simulink model "PMSM_FOC_Average_Inveter"  (R2020b)
settings: Solver=FixedStepAuto  StartTime=0.0  StopTime=10  FixedStep=Fixed_Step_Size  RelTol=1e-3
model workspace (MAT data in the model file):
  wc : Simulink.Parameter (value not decoded)
values from neighbouring files (symbols this model uses):
  Angle = 1.0    [Hall_HSMO_FOC_Data.sldd]    (also in Hall_SMO_FOC_Data.sldd)
  Angle_offset = 0.1985    [Hall_HSMO_FOC_Data.sldd]    (also in Hall_SMO_FOC_Data.sldd)
  Cosine_table = 1.0 0.99999529 0.99999058 0.99998587 0.99998116 0.99996704 0.99995291 0.99993885 0.99992472 0.99990118 0.99987763 0.99985409 0.9998306 0.99979764 0.99976468 0.99973178 0.99969882 0.99965644 0.99961412 0.99957174 0.99952942 0.99947762 0.99942589 0.99937415 0.99932235 0.9992612 0.99920005 0.99913889 0.99907768 0.99900717 0.99893659 0.99886602 0.99879545 0.99871546 0.99863547 0.99855554 0.99847555 0.    [Hall_HSMO_FOC_Data.sldd]    (also in Hall_SMO_FOC_Data.sldd)
  Fixed_Step_Size = 2.5E-5    [Hall_HSMO_FOC_Data.sldd]    (also in Hall_SMO_FOC_Data.sldd = 1.0E-5
  Flux = 0.0109    [G474_FOC_HSMO.sldd]    (also in Hall_HSMO_FOC_Data.sldd = 0.00529276
  FluxWeak_Enable = 0.0    [Hall_HSMO_FOC_Data.sldd]    (also in Hall_SMO_FOC_Data.sldd)
  FluxWeak_Idref_max = 0.0    [Hall_HSMO_FOC_Data.sldd]    (also in Hall_SMO_FOC_Data.sldd)
  FluxWeak_Idref_min = -200.0    [Hall_HSMO_FOC_Data.sldd]    (also in Hall_SMO_FOC_Data.sldd)
  FluxWeak_Ki = 50.0    [Hall_HSMO_FOC_Data.sldd]    (also in Hall_SMO_FOC_Data.sldd)
  FluxWeak_Kp = 1.2    [Hall_HSMO_FOC_Data.sldd]    (also in Hall_SMO_FOC_Data.sldd)
  ID_Ki = 450.0    [Hall_HSMO_FOC_Data.sldd]    (also in Hall_SMO_FOC_Data.sldd = 0.8
  ID_Kp = 0.4    [Hall_HSMO_FOC_Data.sldd]    (also in Hall_SMO_FOC_Data.sldd = 3.2
  IQ_Ki = 450.0    [Hall_HSMO_FOC_Data.sldd]    (also in Hall_SMO_FOC_Data.sldd = 0.32
  IQ_Kp = 0.45    [Hall_HSMO_FOC_Data.sldd]    (also in Hall_SMO_FOC_Data.sldd = 3.3
  Ld = 0.000195185    [G474_FOC_HSMO.sldd]    (also in Hall_HSMO_FOC_Data.sldd = 0.0004
  Lq = 0.000195185    [G474_FOC_HSMO.sldd]    (also in Hall_HSMO_FOC_Data.sldd = 0.00045
  MTPA_id_table = 0.22889 0.23462678 0.23770036 0.2381243 0.23591207 0.23107713 0.2236329 0.21359272 0.20096992 0.18577772 0.16802935 0.14773798 0.12491672 0.099578641 0.071736768 0.041404068 0.0085934745 -0.026682133 -0.064409919 -0.10457709 -0.14717092 -0.1921787 -0.2395878 -0.28938559 -0.34155953 -0.39609709 -0.45298585 -0.51221335 -0.57376724 -0.63763517 -0.70380485 -0.77226412 -0.84300071 -0.91600245 -0.991257    [Hall_HSMO_FOC_Data.sldd]    (also in Hall_SMO_FOC_Data.sldd)
  MTPA_iq_table = -1.0417 -0.16083497 0.71926296 1.5985928 2.4771533 3.3549435 4.2319627 5.1082091 5.9836826 6.8583813 7.732305 8.6054525 9.4778223 10.349415 11.220228 12.090261 12.959513 13.827983 14.69567 15.562573 16.428694 17.294027 18.158575 19.022335 19.885307 20.747492 21.608887 22.469492 23.329306 24.188328 25.046556 25.903992 26.760633 27.616482 28.471533 29.325788 30.179247 31.031908 31.883772 32.734837 3    [Hall_HSMO_FOC_Data.sldd]    (also in Hall_SMO_FOC_Data.sldd)
  MTPA_Te_Max = 800.0    [Hall_HSMO_FOC_Data.sldd]    (also in Hall_SMO_FOC_Data.sldd)
  MTPA_Te_Min = 0.0    [Hall_HSMO_FOC_Data.sldd]    (also in Hall_SMO_FOC_Data.sldd)
  Over_modulation = 0.0    [Hall_HSMO_FOC_Data.sldd]    (also in Hall_SMO_FOC_Data.sldd)
  Pole_Pairs = 2.0    [Hall_HSMO_FOC_Data.sldd]    (also in Hall_SMO_FOC_Data.sldd)
  PWM_Frequency = 10000.0    [Hall_HSMO_FOC_Data.sldd]    (also in Hall_SMO_FOC_Data.sldd)
  Sine_table = 0.0 0.0015339879 0.0030679768 0.0046019657 0.0061359555 0.0076698866 0.0092038177 0.010737749 0.012271681 0.013805497 0.015339312 0.016873131 0.018406944 0.019940587 0.021474229 0.023007872 0.024541514 0.026074925 0.027608337 0.029141748 0.03067516 0.032208283 0.033741407 0.035274528 0.036807653 0.038340431 0.039873205 0.04140598 0.042938754 0.04447113 0.046003502 0.047535874 0.049068246 0.0506001    [Hall_HSMO_FOC_Data.sldd]    (also in Hall_SMO_FOC_Data.sldd)
  Speed_Ki = 0.633    [Hall_HSMO_FOC_Data.sldd]    (also in Hall_SMO_FOC_Data.sldd)
  Speed_Kp = 0.0867    [Hall_HSMO_FOC_Data.sldd]    (also in Hall_SMO_FOC_Data.sldd = 0.0267
  Speed_PI_OutputMax = 6.0    [Hall_HSMO_FOC_Data.sldd]    (also in Hall_SMO_FOC_Data.sldd = 5.0
  Speed_PI_OutputMin = -6.0    [Hall_HSMO_FOC_Data.sldd]    (also in Hall_SMO_FOC_Data.sldd = -5.0
  TorqueMode = 0.0    [Hall_HSMO_FOC_Data.sldd]    (also in Hall_SMO_FOC_Data.sldd)
undefined symbols (not defined in the file or in its folder): DiscIntNeverNeededParam, inverter, sigbuilder_block, SVPWM
libraries: simulink x7, pid_lib x1, mcbplantlib x1, autolibpmsminterior x1
(part 3 of 3)

== stateflow chart PMSM_FOC_Average_Inveter/Motor_Control/Motor_Control_Function/SYM_State_10ms/Traction_SYM ==
  state Drive
    en:
    stSysCtlDes = Drive;
    SYM_Current_State=0;
    state SYM_InvrStM
      en,du:
      state Second_State
        state Init
          en,du:
          flgTranDrvInit=1;
        state DrvInit
          en,du:
          flgTranDrvInitToCal=1;
        state Calibration
          state MoCSop
            en,du:
            stSysCtlDes=MoCSop;
          state SensCalFW
            en,du:
            stSysCtlDes=SensCalFW
          state TestPulse
            en,du:
            stSysCtlDes=TestPulse
          (default) -> MoCSop
          SensCalFW -> TestPulse : [flgTranSnsrCalToTestPls]
          MoCSop -> SensCalFW : [flgTranMoCSOPToSnsrCal]
        state FreeWheel
          en,du:
          stSysCtlDes=FreeWheel;
        state alOffsetCalFW
          en,du:
          stSysCtlDes=alOffsetCalFW;
        state Standby
          en,du:
          stSysCtlDes=Standby;
          SYM_flgRunRea=1;
          Standby -> (junction 246) [order 1]
          (junction 246) -> Standby : [stDrvCtlDes==Run]{flgTranStbToCtrl=1}
        state alOffsetCalAcc
          en,du:
          stSysCtlDes=alOffsetCalAcc;
        state Run
          en,du:
          stSysCtlDes=Run;
          flgTranStbToCtrl=1;
          SYM_flgRunRea=0;
          exit:
          SYM_flgRunRea=1;
          Run -> (junction 243) [order 1]
          (junction 243) -> Run : [stDrvCtlDes==Standby]{flgTranStbToCtrl=0}
        (default) -> Init
        (junction 145) -> Init [order 1] : [~flgStbRea]
        Init -> DrvInit : [flgTranDrvInit]
        FreeWheel -> (junction 145) : [~flgTranToFW]
        (junction 145) -> Standby [order 2] : [flgStbRea]
        DrvInit -> Run [order 3] : [flgTranDrvInitToCal ...
            | &&stDrvCtlDes== Run]
        DrvInit -> Standby [order 2] : [flgTranDrvInitToCal ...
            | &&stDrvCtlDes== Standby]
        DrvInit -> Calibration [order 1] : [flgTranDrvInitToCal ...
            | &&stDrvCtlDes== Calibration]
        Second_State -> FreeWheel [order 1] : [flgTranToFW]
        Calibration -> Run [order 1] : [flgTranMoCSOPToRun ...
            | && stDrvCtlDes== Run ]
        Calibration -> Standby [order 2] : [flgTranCalToStb]
        alOffsetCalFW -> Standby [order 1] : [stDrvCtlDes~=alOffsetCalFW]
        Standby -> alOffsetCalFW [order 2] : [stDrvCtlDes==alOffsetCalFW]
        alOffsetCalFW -> alOffsetCalAcc [order 2] : [stDrvCtlDes==alOffsetCalAcc]
        alOffsetCalAcc -> alOffsetCalFW [order 1] : [stDrvCtlDes==alOffsetCalFW]
        Run -> Standby [order 1] : [~flgTranStbToCtrl]
        Standby -> Run [order 1] : [flgTranStbToCtrl]
        Standby -> alOffsetCalAcc [order 3] : [stDrvCtlDes==alOffsetCalAcc]
        alOffsetCalAcc -> Standby [order 2] : [stDrvCtlDes~=alOffsetCalAcc]
      state Failure
        en,du:
        stSysCtlDes=FreeWheel;
      state Discharge
        en,du:
        stSysCtlDes=Discharge;
      (default) -> Second_State
      Failure -> (junction 145) : [flgTranErrToStb]
      Discharge -> (junction 145) : [~flgTranDcha]
      Second_State -> Failure [order 1] : [flgTranToErr]
      SYM_InvrStM -> Discharge [order 1] : [flgTranDcha]
    state SYM_Invrlnp
      en:SYM_Current_State=10;
      state SYM_Invrlnp_Check
        en:SYM_Current_State=11;
      (default) -> SYM_Invrlnp_Check
    (junction 258) -> Drive
    SYM_Invrlnp -> (junction 258) : [ISC_bT15==0]{flgAllwDrv=0}
    SYM_InvrStM -> (junction 258) [order 1] : [ISC_bT15==0]{flgAllwDrv=0}
    (default) -> SYM_Invrlnp
    SYM_Invrlnp_Check -> SYM_InvrStM : [flgCmpIMsg ...
        | && ISC_UdcLnkFlt>10 ...
        | && ISC_UdcLnkFlt<450 ...
        | && ISC_bT15 ...
        | && stSysCtlDes==Drive]
  state SYM_OperInp
    en,du:
    flgAllwDrv=0;
    SYM_Current_State=SYM_OperInp;
  state PreDrive
    en:
    stSysCtlDes = PreDrive;
    flgAllwDrv=1;
    %tiPreActvTi++;
    SYM_Current_State=PreDrive;
  state PostDrive
    en:
    stSysCtlDes=PostDrive;
    SYM_Current_State=PostDrive;
  state ShutDown
    en:
    stSysCtlDes = ShutDown
    SYM_Current_State=ShutDown;
  PostDrive -> PreDrive : [stSysCtrl==PreDrive]
  (default) -> SYM_OperInp
  PreDrive -> Drive [order 1] : [flgInitRdy&& ...
      | flgAllwDrv&& ...
      | flgPreDrvDne&& ...
      | ISC_bT15&& ...
      | after(10,tick)]
  Drive -> PostDrive : [~flgAllwDrv]
  SYM_OperInp -> PreDrive : [ISC_bT15==1 ...
      | | ISC_UdcLnkFlt>60 ...
      | | ISC_n>500 ...
      | | ISC_Is>50]
  PreDrive -> ShutDown [order 2] : [flgAllwDrv&& ...
      | flgPreDrvEx&& ...
      | after(10,tick)]
  ShutDown -> SYM_OperInp : [ISC_bT15==1 ...
      | | ISC_UdcLnkFlt>60 ...
      | | ISC_n>500 ...
      | | ISC_Is>50]
  data: flgStbRea local boolean; flgTranCalToStb local boolean; flgTranDcha local boolean; flgTranDrvInitToCal local boolean; flgTranErrToStb local boolean; flgTranMoCSOPToRun local boolean; flgTranMoCSOPToSnsrCal local boolean; flgTranSnsrCalToTestPls local boolean; flgTranStbToCtrl local boolean; flgTranToErr local boolean; flgTranToFW local boolean; Cif_stSysCtrl input uint8; ISC_UdcLnkFlt input int16; ISC_Is input int16; ISC_n input int16; ISC_bT15 input boolean; flgPostDrvDne input uint8; flgPreDrvDne input uint8; flgPreDrvEx input uint8; stSysCtrl input uint8; flgInitRdy input boolean; flgCmpIMsg input uint8; stDrvCtlDes input uint8; ISC_stAlRtrOfs input uint8; ISC_stDesAlRtrOfsClb input uint8; MCT_stFrwhl input uint8; SYM_stDcha input uint8; SYM_Current_State output uint8; SYM_stDrvCtrl output uint8; SYM_stGateDrv output uint8; SYM_flgRunRea output uint8; SYM_OperInp constant uint8 =1; PreDrive constant uint8 =2; ShutDown constant uint8 =5; Drive constant uint8 =3; SYM_Invrlnp constant uint8 =17; SYM_InvrStM constant uint8 =18; PostDrive constant uint8 =4; stSysCtlDes local uint8; flgAllwDrv local boolean; flgTranDrvInit local boolean; stHvbCntct input uint8; bReadyHv input uint8; Calibration constant uint8 =6; MoCSop constant uint8 =7; SensCalFW constant uint8 =8; TestPulse constant uint8 =9; Standby constant uint8 =10; Run constant uint8 =11; alOffsetCalFW constant uint8 =12; alOffsetCalAcc constant uint8 =13; Failure constant uint8 =14; FreeWheel constant uint8 =15; Discharge constant uint8 =16
